simulink model "FM"  (R2022a)
settings: Solver=VariableStepAuto  StartTime=0.0  StopTime=9  RelTol=1e-3
InitFcn:
  | fm_init()
StopFcn:
  | fm_plots()
  | fm_play()
libraries: commanapbnd3 x2, commchan3 x1
settings Model: Creator=aliel  LastModifiedBy=aliel

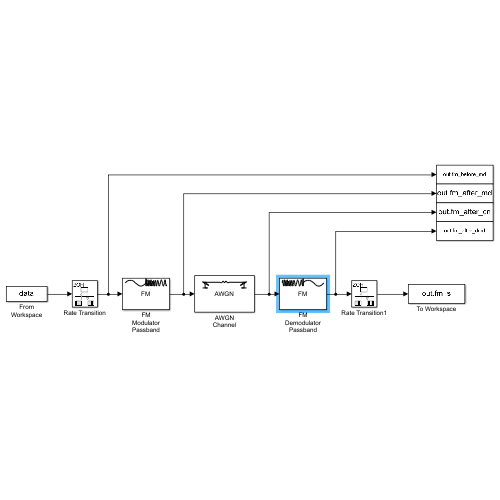
[thumbnail: Simulink's stored preview of the top-level diagram]
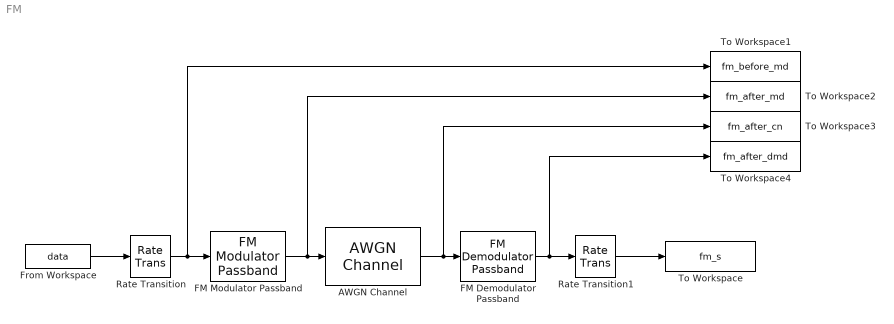
== system FM ==
  AWGN Channel : commchan3/AWGN Channel  InputProcessing=Columns as channels (frame based)  seed=67  noiseMode="Signal to noise ratio  (SNR)"  EbNodB=10  EsNodB=10  SNRdB=150  bitsPerSym=1  Ps=0.5  Tsym=1  variance=1
  FM Demodulator Passband : commanapbnd3/FM Demodulator Passband  Fc=40e3  Ph=0  Kc=2.5e3  Ho=200
      settings: SourceProductBaseCode=CM
  FM Modulator Passband : commanapbnd3/FM Modulator Passband  Fc=40e3  Ph=0  Kc=2.5e3
      settings: SourceProductBaseCode=CM
  From Workspace : FromWorkspace  VariableName=data
  Rate Transition : RateTransition  OutPortSampleTime=1/(8192*15)
  Rate Transition1 : RateTransition  OutPortSampleTime=1/8192
  To Workspace : ToWorkspace  VariableName=fm_s  SampleTime=-1
      settings: Save2DSignal=2-D array (concatenate along first dimension)
  To Workspace1 : ToWorkspace  VariableName=fm_before_md  SampleTime=-1
      settings: Save2DSignal=2-D array (concatenate along first dimension)
  To Workspace2 : ToWorkspace  VariableName=fm_after_md  SampleTime=-1
      settings: Save2DSignal=2-D array (concatenate along first dimension)
  To Workspace3 : ToWorkspace  VariableName=fm_after_cn  SampleTime=-1
      settings: Save2DSignal=2-D array (concatenate along first dimension)
  To Workspace4 : ToWorkspace  VariableName=fm_after_dmd  SampleTime=-1
      settings: Save2DSignal=2-D array (concatenate along first dimension)
  wires:
  AWGN Channel/1 -> To Workspace3/1, FM Demodulator Passband/1
  From Workspace/1 -> Rate Transition/1
  Rate Transition/1 -> To Workspace1/1, FM Modulator Passband/1
  FM Modulator Passband/1 -> To Workspace2/1, AWGN Channel/1
  FM Demodulator Passband/1 -> To Workspace4/1, Rate Transition1/1
  Rate Transition1/1 -> To Workspace/1
